simulink model "Testbed_ClosedLoop"  (R2024b)
settings: Solver=VariableStepAuto  StartTime=0.0  StopTime=tf  RelTol=1e-3
values from neighbouring files (symbols this model uses):
  p1 = linspace(gamma1_min,gamma1_max,10)    [CMG_Testbed_Attitude_Control.m]
  p2 = linspace(gamma2_min,gamma2_max,10)    [CMG_Testbed_Attitude_Control.m]
undefined symbols (not defined in the file or in its folder): K1, K2, K3, K4
libraries: simulink_extras x4, cstblocks x1
settings Model: Creator=lanhi  LastModifiedBy=lanhi

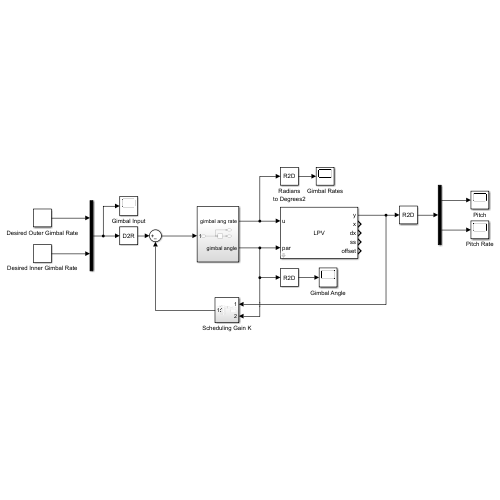
[thumbnail: Simulink's stored preview of the top-level diagram]
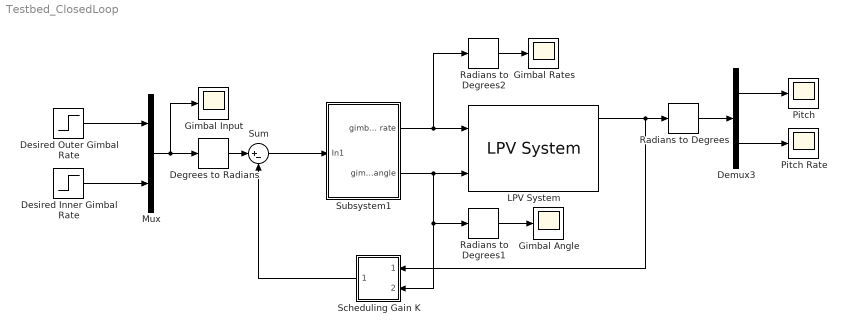
== system Testbed_ClosedLoop ==
  Degrees to Radians : simulink_extras/Transformations/Degrees to Radians
  Demux3 : Demux  Outputs=2
  Desired Inner Gimbal Rate : Step  After=0  SampleTime=0
  Desired Outer Gimbal Rate : Step  After=0  SampleTime=0
  Gimbal Angle : Scope
  Gimbal Input : Scope
  Gimbal Rates : Scope
  LPV System : cstblocks/Linear Parameter Varying/LPV System  sys=ICs  InitialConditionSource=internal  InitialCondition=[deg2rad(45),0]  opSpecOption=Specify offsets as double arrays  uOffset=0  yOffset=0  xOffset=0  opEquilOption=on  dxOffset=0  AFixed=false  BFixed=false  CFixed=false  DFixed=false  uDelayFixed=false  yDelayFixed=false  iDelayFixed=false  sysFixedOption=First model in state-space array  sysFixed=[]  IMethod=Linear  EMethod=Clip  IndexSearch=Binary search  IndexBegin=on  OutputX=on  OutputXdot=on  OutputLTI=on  OutputOP=on  DataType=double  InitBufferSize=1024  FixedBuffer=off  SimMode=Interpreted execution  Offset=struct
  Mux : Mux  Inputs=2
  Pitch : Scope
  Pitch Rate : Scope
  Radians to Degrees : simulink_extras/Transformations/Radians to Degrees
  Radians to Degrees1 : simulink_extras/Transformations/Radians to Degrees
  Radians to Degrees2 : simulink_extras/Transformations/Radians to Degrees
  Scheduling Gain K : Subsystem
  Subsystem1 : Subsystem
  Sum : Sum  Inputs=|+-
  wires:
  Subsystem1/2(gimbal angle) -> Scheduling Gain K/2(In2), Radians to Degrees1/1, LPV System/2
  Radians to Degrees/1 -> Demux3/1
  Radians to Degrees1/1 -> Gimbal Angle/1
  Desired Outer Gimbal Rate/1 -> Mux/1
  Desired Inner Gimbal Rate/1 -> Mux/2
  Mux/1 -> Degrees to Radians/1, Gimbal Input/1
  Degrees to Radians/1 -> Sum/1
  LPV System/1 -> Scheduling Gain K/1(In1), Radians to Degrees/1
  Scheduling Gain K/1(Out1) -> Sum/2
  Sum/1 -> Subsystem1/1(In1)
  Subsystem1/1(gimbal ang rate) -> Radians to Degrees2/1, LPV System/1
  Demux3/1 -> Pitch/1
  Demux3/2 -> Pitch Rate/1
  Radians to Degrees2/1 -> Gimbal Rates/1

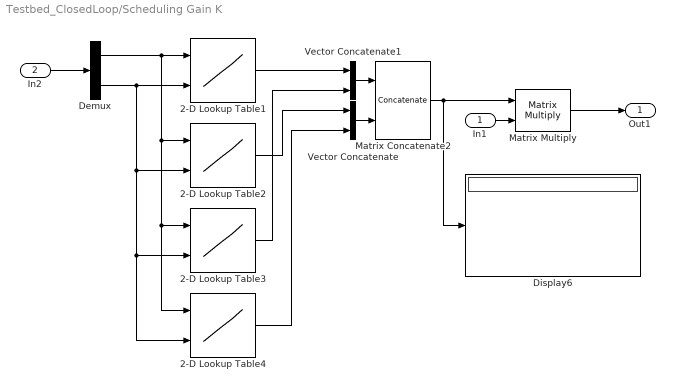
== system Testbed_ClosedLoop/Scheduling Gain K ==
  In1 : Inport
  In2 : Inport  Port=2
  2-D Lookup Table1 : Lookup_n-D  BreakpointsForDimension1=p1  BreakpointsForDimension2=p2  Table=K1  InternalRulePriority=Speed  RndMeth=Simplest
      settings: InputPortMap=u0,u1
  2-D Lookup Table2 : Lookup_n-D  BreakpointsForDimension1=p1  BreakpointsForDimension2=p2  Table=K2  InternalRulePriority=Speed  RndMeth=Simplest
      settings: InputPortMap=u0,u1
  2-D Lookup Table3 : Lookup_n-D  BreakpointsForDimension1=p1  BreakpointsForDimension2=p2  Table=K3  InternalRulePriority=Speed  RndMeth=Simplest
      settings: InputPortMap=u0,u1
  2-D Lookup Table4 : Lookup_n-D  BreakpointsForDimension1=p1  BreakpointsForDimension2=p2  Table=K4  InternalRulePriority=Speed  RndMeth=Simplest
      settings: InputPortMap=u0,u1
  Demux : Demux  Outputs=2
  Display6 : Display
  Matrix Concatenate2 : Concatenate  Mode=Multidimensional array  ConcatenateDimension=2
  Matrix Multiply : Product  Multiplication=Matrix(*)
  Vector Concatenate : Concatenate
  Vector Concatenate1 : Concatenate
  Out1 : Outport
  wires:
  Demux/2 -> 2-D Lookup Table4/2, 2-D Lookup Table3/2, 2-D Lookup Table2/2, 2-D Lookup Table1/2
  In1/1 -> Matrix Multiply/2
  2-D Lookup Table3/1 -> Vector Concatenate1/2
  Vector Concatenate/1 -> Matrix Concatenate2/2
  2-D Lookup Table4/1 -> Vector Concatenate/2
  2-D Lookup Table1/1 -> Vector Concatenate1/1
  Matrix Concatenate2/1 -> Display6/1, Matrix Multiply/1
  2-D Lookup Table2/1 -> Vector Concatenate/1
  Demux/1 -> 2-D Lookup Table4/1, 2-D Lookup Table3/1, 2-D Lookup Table2/1, 2-D Lookup Table1/1
  Vector Concatenate1/1 -> Matrix Concatenate2/1
  In2/1 -> Demux/1
  Matrix Multiply/1 -> Out1/1

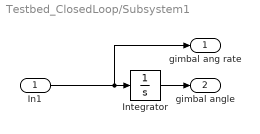
== system Testbed_ClosedLoop/Subsystem1 ==
  In1 : Inport
  Integrator : Integrator  InitialCondition=[0,0]
  gimbal ang rate : Outport
  gimbal angle : Outport  Port=2
  wires:
  Integrator/1 -> gimbal angle/1
  In1/1 -> gimbal ang rate/1, Integrator/1
